simulink model "Guia_9_Ejercicio_3_simulink"  (R2016a)
settings: Solver=VariableStepAuto  StartTime=0.0  StopTime=10.0  RelTol=1e-3
settings Model: Creator=Abel  LastModifiedBy=Abel

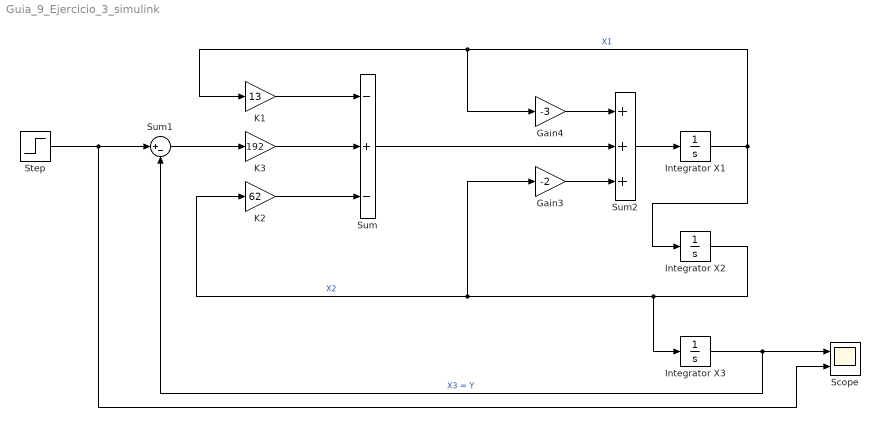
== system Guia_9_Ejercicio_3_simulink ==
  Gain3 : Gain  Gain=-2
  Gain4 : Gain  Gain=-3
  Integrator X1 : Integrator
  Integrator X2 : Integrator
  Integrator X3 : Integrator
  K1 : Gain  Gain=13
  K2 : Gain  Gain=62
  K3 : Gain  Gain=192
  Scope : Scope  NumInputPorts=2
  Step : Step  SampleTime=0
  Sum : Sum  Inputs=-+-
  Sum1 : Sum  Inputs=|+-
  Sum2 : Sum  Inputs=+++
  wires:
  K2/1 -> Sum/3
  Step/1 -> Scope/2, Sum1/1
  Sum2/1 -> Integrator X1/1
  Gain4/1 -> Sum2/1
  Integrator X1/1 -> Gain4/1, K1/1, Integrator X2/1  "X1"
  Integrator X2/1 -> Integrator X3/1, K2/1, Gain3/1  "X2"
  Integrator X3/1 -> Sum1/2, Scope/1  "X3 = Y"
  Gain3/1 -> Sum2/3
  Sum/1 -> Sum2/2
  K1/1 -> Sum/1
  K3/1 -> Sum/2
  Sum1/1 -> K3/1
